simulink model "Gesamt"  (R2015b)
settings: Solver=ode3  SolverMode=SingleTasking  StartTime=0.0  StopTime=inf  RelTol=1e-3
InitFcn:
  | Reglerauslegung
values from neighbouring files (symbols this model uses):
  aMax = 498    [Reglerauslegung.m]
  aMaxPsi = 1    [Reglerauslegung.m]
  Blindzeit = 25    [Reglerauslegung.m]
  dt = 0.005    [Reglerauslegung.m]
  K1 = place(AI1,BI1,pWunschI1)    [Reglerauslegung.m]
  K2 = place(A2,B2,pWunsch2)    [Reglerauslegung.m]
  K3 = place(A3,B3,pWunsch3)    [Reglerauslegung.m]
  Kx = 0.9575    [Reglerauslegung.m]
  Ky = 0.9575    [Reglerauslegung.m]
  Tx = 1/4.1668    (= 0.239992320246)    [Reglerauslegung.m]
  Ty = 1/4.1668    (= 0.239992320246)    [Reglerauslegung.m]
  vMax = 403    [Reglerauslegung.m]
  vMaxPsi = 3    [Reglerauslegung.m]
undefined symbols (not defined in the file or in its folder): sigbuilder_block
libraries: simulink x5, xpcutilitieslib x1
(part 2 of 3)

== stateflow chart Gesamt/Bahnplanung1/Kommunikation_mit_GW1_3 ==
  settings: updateMethod=DISCRETE  sampleTime=dt
  state KommunikationGW3
    state Transportbereich
      entry:Transportbereich=1,
      Fertigungsbereich=0,
      Bereich_Verlassen=0,
      Status=1;
    state Fertigungsbereich
      entry:Transportbereich=0,
      Fertigungsbereich=1;
      state RFID_einchecken
        entry:Zielposition=Ziel-mod(Ziel,10)+3,
        Aktion_an_Position=Aktion_Warten,
        Status=2;
      state Startpunkt
        entry: Zielposition=Ziel-mod(Ziel,10);
        Aktion_an_Position=Aktion_Warten,
        Status=1;
      state Warten1
      state Warten
        during: Bereich_Verlassen=1,
      state Position_anfahren
        entry:Zielposition=Ziel,
        Status=1,
        if Werkstueck==0
        Aktion_an_Position=Aktion_Aufnehmen;
        else
        Aktion_an_Position=Aktion_Ablegen;
        end
      state Bereich_verlassen_vorne1
        entry:Zielposition=Ziel-mod(Ziel,10),
        Aktion_an_Position=Aktion_Warten,
        Status=1;
      state Bereich_verlassen_hinten
        entry:Zielposition=Ziel-mod(Ziel,10)+4,
        Aktion_an_Position=Aktion_Warten,
        Status=1;
      state Bereich_verlassen
        entry:
        ersterFifo=floor(floor(Ziel/10)/2)*3+2*mod(floor(Ziel/10),2)+1;
        Aktion_an_Position=Aktion_Warten,
      state RFID_auschecken
        entry:Zielposition=Ziel-mod(Ziel,10)+3,
        Aktion_an_Position=Aktion_Warten,
        Status=3;
      state Warten2
      Startpunkt -> RFID_einchecken [order 1] : [Ziel_anfordern==1 & Werkstueck==1]
      (default) -> Startpunkt
      RFID_einchecken -> Warten1 : [Ziel_anfordern==1 ]
      Startpunkt -> Position_anfahren [order 2] : [Ziel_anfordern==1 & Werkstueck==0]
      Warten1 -> Position_anfahren : [RFID_Anmeldung==1]
      Bereich_verlassen_vorne1 -> Warten : [Ziel_anfordern==1]
      Bereich_verlassen_hinten -> Warten : [Ziel_anfordern==1]
      Position_anfahren -> Bereich_verlassen [order 2] : [Ziel_anfordern==1 & (Aktion_an_Position==Aktion_Ablegen)]
      Position_anfahren -> RFID_auschecken [order 1] : [Ziel_anfordern==1 & (Aktion_an_Position==Aktion_Aufnehmen)]
      Bereich_verlassen -> Bereich_verlassen_vorne1 [order 1] : [FifoArray(ersterFifo)==0]
      Bereich_verlassen -> Bereich_verlassen_hinten [order 2]
      Warten2 -> Bereich_verlassen : [RFID_Abmeldung==1]
      RFID_auschecken -> Warten2 : [Ziel_anfordern==1]
    state Warten3
    state Ladestationanfahren
      entry:Transportbereich=0,
      Fertigungsbereich=1,
      Status=1;
    (default) -> Transportbereich
    Transportbereich -> Fertigungsbereich [order 1] : [(ZielStation_Erreicht==1) & (floor(Ziel/10)<=7)]
    Warten3 -> Transportbereich
    Transportbereich -> Ladestationanfahren [order 2] : [(ZielStation_Erreicht==1) & (floor(Ziel/10)>7)]
    Fertigungsbereich -> Warten3 : [Bereich_Verlassen==1]
  data: Transportbereich output; Fertigungsbereich output; Ziel input; Zielposition output; Aktion_an_Position output double; Aktion_Warten local double =0; Aktion_Aufnehmen local double =1; Aktion_Ablegen local double =2; Werkstueck input double; Bereich_Verlassen local; Status output; FifoArray input; ersterFifo local double; Ziel_anfordern input; ZielStation_Erreicht input double; RFID_Anmeldung input; RFID_Abmeldung input

== matlab function Gesamt/Bahnplanung1/Positionen_Robotinos_Filtern ==
  data: UDPDaten input; RobPos output; RobotinoID input; StoerPos output size=[1 15]; altePos input size=[1 15]; altePos1 output size=[1 15]
function [RobPos,StoerPos,altePos1]      = fcn(UDPDaten , RobotinoID, altePos)
StoerPos=zeros([1 15]);
RobPos=zeros([1 3]);
altePos1=zeros([1 15]);
%     case 5
%         RobPos(1:3) = UDPDaten(13:15);
%         StoerPos(1:12)=UDPDaten(1:12);
%Positionmerken
for x=0:4
    temp=abs(UDPDaten((x*3)+1:(x*3)+3));
    test=sum(temp);
    if(test==0)
     altePos1((x*3)+1:(x*3)+3)=altePos((x*3)+1:(x*3)+3);
    else
     altePos1((x*3)+1:(x*3)+3)=UDPDaten((x*3)+1:(x*3)+3);
    end
end

 if RobotinoID == 4
        RobPos(1:3) = altePos1(10:12);
        StoerPos(1:9)=altePos1(1:9);
        %  StoerPos(10:12)=UDPDaten(13:15);
    elseif RobotinoID == 3
        RobPos(1:3) = altePos1(7:9);
        StoerPos(1:6)=altePos1(1:6);
        StoerPos(7:9)=altePos1(10:12);%      StoerPos(7:12)=UDPDaten(10:15);
    elseif RobotinoID == 2
        RobPos(1:3) = altePos1(4:6);
        StoerPos(1:3)=altePos1(1:3);
        StoerPos(4:9)=altePos1(7:12);%     StoerPos(4:12)=UDPDaten(7:15);
        elseif RobotinoID == 1
        RobPos(1:3) = altePos1(1:3);
        StoerPos(1:9)=altePos1(4:12);%     StoerPos(1:12)=UDPDaten(4:15);
end

== matlab function Gesamt/Bahnplanung1/Trafo ==
  data: Vektor input; V_RobX output; Winkel input; V_RobY output
function [V_RobX, V_RobY]= fcn(Vektor,Winkel)
V_RobX=(cos(Winkel)*Vektor(1)+sin(Winkel)*Vektor(2));
V_RobY=(cos(Winkel)*Vektor(2)-sin(Winkel)*Vektor(1));

== matlab function Gesamt/Bahnplanung1/Vektorberechnung/AusweichVektorBerechnung ==
  data: Vektor_In input; Vektor output; Ausweichwert input; Zone input; RobotinoPos input; ZielPos input
function Vektor  = fcn(Vektor_In,Ausweichwert,Zone,RobotinoPos,ZielPos)
Vektor=zeros([1 2]);
%Ausweichmanöver
Distanz=sqrt((RobotinoPos(1)-ZielPos(1))^2+(RobotinoPos(2)-ZielPos(2))^2);
K=3;
AVX=zeros([1 4]);
AVY=zeros([1 4]);
 for x=1:4
 AVX(x)=-K*Ausweichwert(2,x)*cos(Ausweichwert(1,x));
 AVY(x)=-K*Ausweichwert(2,x)*sin(Ausweichwert(1,x));
 end
if (Zone==0) && ((Distanz > 300)&&(RobotinoPos(2)> 500)&&(RobotinoPos(1)> 500))
 VektorX=Vektor_In(1)+sum(AVX);
 VektorY=Vektor_In(2)+sum(AVY);
else
 VektorX=Vektor_In(1);
 VektorY=Vektor_In(2);
end

%Bremsen vor dem Ziel

MaxDis=1000;
if Distanz > MaxDis
Vektor(1) = VektorX;
Vektor(2) = VektorY;
else
Vektor(1) = VektorX*Distanz/MaxDis;
Vektor(2) = VektorY*Distanz/MaxDis;  
end

end

== matlab function Gesamt/Bahnplanung1/Vektorberechnung/Ausweichmanoever ==
  data: RobotinoPos input; StoerPos input; Vektor input; Ausweich output
function Ausweich  = fcn(RobotinoPos, StoerPos, Vektor)
Abstand=zeros([2 4]);
Ausweich=zeros([2 4]);%Zeile1 =Richtung(winkel in Rad) Zeile2=Intensität
for i=1:4
    Abstand(1,i)=-RobotinoPos(1)+StoerPos(1+((i-1)*3));
    Abstand(2,i)=-RobotinoPos(2)+StoerPos(2+((i-1)*3));
    Hyp=sqrt(Abstand(1,i)^2+Abstand(2,i)^2);
    if Hyp <=1000
        if Abstand(1,i) >= 0
             Ausweich(1,i)=+asin(Abstand(2,i)/Hyp)-pi/2;
        else
            Ausweich(1,i)=-asin(Abstand(2,i)/Hyp)+pi/2;
        end
        HypZiel=sqrt(Vektor(1)^2+Vektor(2)^2);
         if Vektor(1) >= 0
            Fahrwinkel=+asin(Vektor(2)/HypZiel);
        else
            Fahrwinkel=-asin(Vektor(2)/HypZiel)+pi;
        end
        if abs(Fahrwinkel-(Ausweich(1,i)+pi/2))<=pi
            if((Fahrwinkel-(Ausweich(1,i)+pi/2)) <= pi/6) && ((Fahrwinkel-(Ausweich(1,i)+pi/2))  >= -pi/6)
            Ausweich(2,i)=1;
             else
           Ausweich(2,i)=0; 
            end
        else
            if((2*pi)-abs(Fahrwinkel-(Ausweich(1,i)+pi/2)) <= pi/6) 
            Ausweich(2,i)=1;
             else
           Ausweich(2,i)=0; 
            end
        end
        if (abs(Fahrwinkel)>pi/2) && (RobotinoPos(2)>1900)
             if abs(Fahrwinkel-(Ausweich(1,i)+pi/2))<=pi
            if((Fahrwinkel-(Ausweich(1,i)+pi/2)) <= pi/6) && ((Fahrwinkel-(Ausweich(1,i)+pi/2))  >= -pi/6)
            Ausweich(2,i)=-1;
             else
           Ausweich(2,i)=0; 
            end
        else
            if((2*pi)-abs(Fahrwinkel-(Ausweich(1,i)+pi/2)) <= pi/6) 
            Ausweich(2,i)=-1;
             else
           Ausweich(2,i)=0; 
            end
        end
        end
%         if (Vektor(2)~=0) && (sin(Ausweich(1,i)+pi/2)~=0)
%             Ausweich(2,i)=Vektor(2)/sin(Ausweich(1,i)+pi/2);
%         elseif (Vektor(1)~=0)&&(cos(Ausweich(1,i)+pi/2)~=0)
%              Ausweich(2,i)=Vektor(1)/cos(Ausweich(1,i)+pi/2);
%         else
%              Ausweich(2,i)=0;
%         end
    else
        Ausweich(1,i)=0;
        Ausweich(2,i)=0;
    end
    if StoerPos(2+((i-1)*3))<300
        Ausweich(2,i)=0;
    end
end

== matlab function Gesamt/Bahnplanung1/Vektorberechnung/FahrendeRobotinosErkennen ==
  data: Stoerpos input; Robotinofaehrt output; Stoeralt input
function Robotinofaehrt = fcn(Stoerpos,Stoeralt)
Robotinofaehrt=zeros([1 4]);
for x=1:4
    if (abs(Stoeralt(1+(3*(x-1)))-Stoerpos(1+(3*(x-1)))) >= 10) && (abs(Stoeralt(2+(3*(x-1)))-Stoerpos(2+(3*(x-1)))) >= 10)
        Robotinofaehrt(x)=1;
    else
        Robotinofaehrt(x)=0;
    end
end

== matlab function Gesamt/Bahnplanung1/Vektorberechnung/IR_Daten_Erfassen ==
  data: RobotinoDaten input; IRWerte output; RobPos input
function IRWerte = fcn(RobotinoDaten,RobPos)
IRWerte=zeros([2 9]);
IRDaten=zeros([1 9]);
IRDaten=RobotinoDaten(6:14);

for x=1:9
    if  (isnan(IRDaten(x))==0) && (IRDaten(x) <= 120)
    IRWerte(1,x)=cos(((x-1)*40*pi/180)+RobPos(3))*(IRDaten(x)+200)+RobPos(1);
    IRWerte(2,x)=sin(((x-1)*40*pi/180)+RobPos(3))*(IRDaten(x)+200)+RobPos(2);
    else
    IRWerte(1,x)=NaN;
    IRWerte(2,x)=NaN;
    end
end

== matlab function Gesamt/Bahnplanung1/Vektorberechnung/Vektorberechnung ==
  data: ZielPos input; Vektor output; RobotinoPos input; StoerPos input; IRWerte input; Zone output; RobotinoFaehrt input; AlteZone input
function [Vektor,Zone] = fcn(ZielPos, RobotinoPos, StoerPos, IRWerte,RobotinoFaehrt,AlteZone)
Stationen=[1103,2308,3507,4694,6300,6300;
            2832,2832,2832,2832,2608,3085;];
Vektor=zeros([1 2]);
%Stationen Einflussvektor
K=400;
sigma=187;
SVX=zeros([1 6]);
SVY=zeros([1 6]);
for x=1:4
SVX(x)= -K*exp(-((RobotinoPos(1)-Stationen(1,x))^2+(RobotinoPos(2)-Stationen(2,x))^2)/(2*(sigma^2)))*((RobotinoPos(1)-Stationen(1,x))/(sigma^2));
SVY(x)= -K*exp(-((RobotinoPos(1)-Stationen(1,x))^2+(RobotinoPos(2)-Stationen(2,x))^2)/(2*(sigma^2)))*((RobotinoPos(2)-Stationen(2,x))/(sigma^2));
end
K=300;
sigma=100; %% mal schauen ob so gut
for x=5:6
SVX(x)= -K*exp(-((RobotinoPos(1)-Stationen(1,x))^2+(RobotinoPos(2)-Stationen(2,x))^2)/(2*(sigma^2)))*((RobotinoPos(1)-Stationen(1,x))/(sigma^2));
SVY(x)= -K*exp(-((RobotinoPos(1)-Stationen(1,x))^2+(RobotinoPos(2)-Stationen(2,x))^2)/(2*(sigma^2)))*((RobotinoPos(2)-Stationen(2,x))/(sigma^2));
end
%Zielvektor
K=0.5;%=0.3;

ZVX = K*(RobotinoPos(1)-ZielPos(1))/sqrt((RobotinoPos(1)-ZielPos(1))^2 +(RobotinoPos(2)-ZielPos(2))^2);
ZVY = K*(RobotinoPos(2)-ZielPos(2))/sqrt((RobotinoPos(1)-ZielPos(1))^2 +(RobotinoPos(2)-ZielPos(2))^2);

%Robtino Stoervektoren
%K=25 im Fifo

RVX=zeros([1 4]);
RVY=zeros([1 4]);
for x=1:4
if (RobotinoFaehrt(x) == 1) && (RobotinoPos(2)> 500)
K=1000;%K=100;
sigma=225;
elseif (RobotinoPos(2)> 2500)
K=500;
sigma=180;
elseif (RobotinoPos(2)< 2500)
K=700;
sigma=180;
end
RVX(x)=-K*exp(-((RobotinoPos(1)-StoerPos((x*3)-2))^2+(RobotinoPos(2)-StoerPos((x*3)-1))^2)/(2*(sigma^2)))*((RobotinoPos(1)-StoerPos((x*3)-2))/(sigma^2));
RVY(x)=-K*exp(-((RobotinoPos(1)-StoerPos((x*3)-2))^2+(RobotinoPos(2)-StoerPos((x*3)-1))^2)/(2*(sigma^2)))*((RobotinoPos(2)-StoerPos((x*3)-1))/(sigma^2));
end

%Infrarot Einflussvektor
K=500;
sigma=250;
IRVX=zeros([1 9]);
IRVY=zeros([1 9]);
for x=1:9
    if(isnan(IRWerte(1,x))==0)||(isnan(IRWerte(2,x))==0)
       if (RobotinoPos(2)> 500)
    IRVX(x)=-K*exp(-((RobotinoPos(1)-IRWerte(1,x))^2+(RobotinoPos(2)-IRWerte(2,x))^2)/(2*(sigma^2)))*((RobotinoPos(1)-IRWerte(1,x))/(sigma^2));
    IRVY(x)=-K*exp(-((RobotinoPos(1)-IRWerte(1,x))^2+(RobotinoPos(2)-IRWerte(2,x))^2)/(2*(sigma^2)))*((RobotinoPos(2)-IRWerte(2,x))/(sigma^2));
       else
    IRVX=0;
    IRVY=0;
       end
    else
    IRVX(x)=0;
    IRVY(x)=0;
    end
end


 
K=0.4; %Steigung der schrägen
x=RobotinoPos(1);
y=RobotinoPos(2);
x_test=0;
y_test=0;
VektorX=0;
VektorY=0;

 if (x >601) && (x<=5301) && (y>2501) && (y<=3201)
    Zone=4;
elseif (x >2751) && (x<=5501) && (y>3201)
    Zone=1;
elseif (x > 601) && (x<=2751) && (y>3201)
    Zone=2;
 elseif (x<=601) && (y>2501)
     Zone=3;  
 elseif (x >5001) && (y>2501) && (AlteZone==1 || AlteZone==5)
     Zone=5;
 else
     Zone=0;
 end

KE=1000;
sigma=50;
Parabel=1000;
 if Zone == 0 % Fahrbereich
     if (x <= 5500) && (y <= 2500)
         x_test=(1/sigma)*KE*exp(-x/sigma);
         y_test=(-1/sigma)*KE*exp((y-2500)/sigma);
     elseif (x > 5500) && (y <= 2500)
         x_test=(1/sigma)*KE*exp((-(x-5500)+(y-2500))/sigma);
         y_test=(-1/sigma)*KE*exp((-(x-5500)+(y-2500))/sigma);
     elseif (x > 5500) && (y > 2500)
         x_test=(1/sigma)*KE*exp(-(x-5500)/sigma);
         y_test=(-1/sigma)*KE*exp((y-3600)/sigma);
     end
 MVX=x_test+(-1/sigma)*KE*exp((x-7000)/sigma);
 MVY=y_test+(1/sigma)*KE*exp(-y/sigma);
 
 VektorX=sum(SVX(5:6))+sum(RVX)+ZVX+sum(IRVX)-MVX;
 VektorY=sum(SVY(5:6))+sum(RVY)+ZVY+sum(IRVY)-MVY;
 elseif Zone == 1 %Rinne nach rechts weg
     MVX=K; %Konstante Steigung
     MVY=-2*(y-3500)/Parabel; % Parabel abgeleitet
 VektorX=sum(RVX)-MVX;
 VektorY=sum(RVY)-MVY;
 elseif Zone == 2 %Rinne nach links weg
     MVX=-K; %Konstante Steigung
     MVY=-2*(y-3500)/Parabel; % Parabel abgeleitet
      VektorX=sum(RVX)-MVX;
      VektorY=sum(RVY)-MVY;
 elseif Zone == 3 %Rinne nach unten weg
     MVX=-2*(x-300)/Parabel; %Konstante Steigung
     MVY=-K; % Parabel abgeleitet
     VektorX=sum(RVX)+sum(IRVX)-MVX;
     VektorY=sum(RVY)+sum(IRVY)-MVY;
 elseif Zone == 5 %Rinne vorne weg
     MVX=-2*(x-5500)/Parabel; %Konstante Steigung
     MVY=-K; % Parabel abgeleitet
     VektorX=sum(RVX)+sum(IRVX)-MVX;
     VektorY=sum(RVY)+sum(IRVY)-MVY;
 else 
     MVX=0;
     MVY=K;
      VektorX=sum(RVX)+sum(SVX(1:4))-MVX;
      VektorY=sum(RVY)+sum(SVY(1:4))-MVY;
 end  
      Vektor(1)=VektorX;
      Vektor(2)=VektorY;
 end

== matlab function Gesamt/Bahnplanung1/Fifo Steuerung/Globale Markierung1 ==
  data: Robbi input; FifoArray input; FifoArray1 output; StationArray1 output; LadeArray input; LadeArray1 output
function [FifoArray1,StationArray1,LadeArray1]= fcn(Robbi,FifoArray,LadeArray)
X=zeros([1 4]);
Y=zeros([1 4]);
X=[Robbi(1) Robbi(4) Robbi(7) Robbi(10)];
Y=[Robbi(2) Robbi(5) Robbi(8) Robbi(11)];
FifoArray1=zeros([1 12]);
FifoArray1=FifoArray(1:12);
StationArray1=zeros([1 8]);
LadeArray1=zeros([1 2]);
LadeArray1=LadeArray(1:2);
N=zeros([1 4]);
S=zeros([1 4]);
L=zeros([1 4]);
for n= 1 : 1 : 4
    L(n)=round((Y(n)-2592)/500)+1;
    N(n)=round((X(n)-703)/400)+1;   % Berechnung in welchem Fifo der Roboter sich befindet
    S(n)=round((X(n)-900)/560)+1;   %Berechnung in welcher Station der Roboter sich befindet
     if (X(n)<=6000 || X(n)>6500)
        for i=1:2
            if LadeArray1(i)==n
                LadeArray1(i)=0;
            end
        end
     end
    if (X(n)>6000 && X(n)<=6500 && Y(n)>2300 && Y(n)<=3300)
        LadeArray1(L(n))=n;
    end  
   
    for i=1:8
          if StationArray1(i)==n
                StationArray1(i)=0;
          end
    end
    if (Y(n)>2100 && Y(n)<3300 && X(n)<5100) && S(n)<=8 && S(n)>0
         for i=1:12
            if FifoArray1(i)==n
                FifoArray1(i)=0;
            end
         end
       
        StationArray1(S(n))=n;
        
    elseif (Y(n)<450 && (X(n)>100 && X(n)<5250)&& N(n)<=12 && N(n)>0)
        for i=1:12
            if FifoArray1(i)==n
                FifoArray1(i)=0;
            end
        end
            FifoArray1(N(n))=n;
           
    elseif (X(n)>6000&& Y(n)<2000)
        for i=1:12
            if FifoArray1(i)==n
                FifoArray1(i)=0;
            end
        end
    end
    end
end

== matlab function Gesamt/Bahnplanung1/Vektorbrbegrenzungberchnen1 ==
  data: Vektor_In input; Vektor output; Transportbereich_aktiv input; RobPos input; FilterIN input; Filter output
function [Vektor,Filter] = fcn(Vektor_In,Transportbereich_aktiv,RobPos,FilterIN)
Vektor=zeros([1 2]);
Filter=zeros([100 2]);
if (Transportbereich_aktiv==1) && (RobPos(1)>=0) && (RobPos(2)>=0)
    

 Filter(1,1)=Vektor_In(1);
 Filter(1,2)=Vektor_In(2);
 for x=1:99
     Filter(x+1,1)=FilterIN(x,1);
     Filter(x+1,2)=FilterIN(x,2);     
 end
 Vektor(1) =sum(Filter(:,1))/100;
 Vektor(2) =sum(Filter(:,2))/100;
 
 %Vektor(1) = Vektor_In(1);
 %Vektor(2) = Vektor_In(2);

if (RobPos(2)<500)||(RobPos(2)>2300)
    for x=1:2
    K=0.3; %Begrenzung langsame Zone
        if  Vektor(x)> K
            Vektor(x) = K;
        elseif Vektor(x) <-K
            Vektor(x)=-K;
        end
    end
else
    for x=1:2
    K=0.5; %Begrenzung schnelle Zone
        if  Vektor(x)> K
            Vektor(x) = K;
        elseif Vektor(x) <-K
            Vektor(x)=-K;
        end
    end
end
end

== matlab function Gesamt/Regelung1/Kalman1 ==
  data: vxZustand input; vyZustand input; vPsiZustand input; PsiZustand input; xZustand input; yZustand input; enable input; dt parameter; vx output; vy output; vpsi output; pospsi output; posx output; posy output; enableBeob output; Blindzeit parameter
function [vx,vy,vpsi,pospsi,posx,posy,enableBeob] = fcn(vxZustand,vyZustand,vPsiZustand,PsiZustand,xZustand,yZustand,enable,dt,Blindzeit)

persistent A H Q RPosX RPosY RPosPsi 
persistent x P
persistent firstRun found counter
QVelX = 0.01;
QVelY = 0.01;
QVelPsi = 0.01;
QPosX = 0.01;
QPosY = 0.01;
QPosPsi = 0.1;
if isempty(firstRun)
found = 0;
x = [0; 0; 0; 0; 2000; 1600];
    

A= [1       0       0       0       0       0;
    0       1       0       0       0       0;
    0       0       1       0       0       0;
    0       0       dt      1       0       0;
    dt      0       0       0       1       0;
    0       dt      0       0       0       1];
    
H = [0 0 0 1 0 0;
     0 0 0 0 1 0;
     0 0 0 0 0 1];

Q = [QVelX       0       0       0       0       0;
     0       QVelY       0       0       0       0;
     0          0       QVelPsi    0       0       0;
     0          0       0       QPosX    0       0;
     0          0       0       0       QPosY    0;
     0          0       0       0       0    QPosPsi];
   
  RPosX = 0.340050836575258;
  RPosY =0.684587581598845;
  RPosPsi=5.754253525875726e-05;

  P =  [1       0       0       0       0       0;
        0       1       0       0       0       0;
        0       0       1       0       0       0;
        0       0       0       1000       0       0;
        0       0       0       0       1000       0;
        0       0       0       0       0       1000];
  
  firstRun = 1; 
  counter = 0;
end


x =[vxZustand ; vyZustand; vPsiZustand;x(4:end,1)];

x = A*x;  
P = A*P*A' + Q;  
counter = counter+1;
dist=0;
Rnow=[RPosX 0 0; 0 RPosY 0; 0 0 RPosPsi];
if enable == 1
    z = [PsiZustand;xZustand;yZustand];
    % Reduzierung der Glaubwürdigkeit bei weit entfernten Messungen
    dist = sqrt(abs(z(2)-x(5))^2 + abs(z(3)-x(6))^2);
    counter =0;
    
%     if dist > 150
%         Rnow = 0;
%         found = 0;
%     elseif dist > 100
%         Rnow = 0.3;
%         found = 0;
%     elseif dist > 20
%         Rnow = 0.2;
%         found = 1;
%     elseif dist < 20
%         found =1;
%         Rnow = 0.5;
%     else 
%         Rnow = R;
%     end

%     if dist > 500
%         Rnow = 0;
%         found = 0;
%     elseif dist > 100
%         Rnow = 0;
%         found = 0;
%     elseif dist > 20
%         Rnow = 0;
%         found = 1;
%     elseif dist < 20
%         found =1;
%         Rnow = 0;
%     else 
%         Rnow = R;
%     end

%     if dist > 500
%         Rnow = eye(3,3)*0;
%         found = 0;
%     elseif dist > 100
%         Rnow=[RPosX-0.1 0 0; 0 RPosY-0.1 0; 0 0 RPosPsi-0.01];
%         found = 0;
%     elseif dist > 20
%         Rnow=[RPosX-0.01 0 0; 0 RPosY-0.01 0; 0 0 RPosPsi];
%         found = 1;
%     else 
%         found = 1;
%         Rnow=[RPosX 0 0; 0 RPosY 0; 0 0 RPosPsi];
%     end
    if dist > 20
        found = 1;
    end
    K =    P*H'*inv(H*P*H' + Rnow); 

    x = x + K*(z - H*x);

    P = P - K*H*P;
end
if counter>= (Blindzeit/dt)
    found = 0;
end
enableBeob = found;

vx      = x(1);
vy      = x(2);
vpsi    = x(3);
pospsi  = x(4);
posx    = x(5);
posy    = x(6);

== matlab function Gesamt/Regelung1/Bereichswaehler ==
  data: modus output; transportbereich input; enable output; fertigungsbereich input
function [modus, enable] = fcn(transportbereich, fertigungsbereich)

enable = false;
modus = 0;

if fertigungsbereich == 1 && transportbereich == 0
    enable = true;
    modus = 1;
end
    
if fertigungsbereich == 0 && transportbereich == 1
    enable = true;
    modus = 0;
end

== matlab function Gesamt/Regelung1/NewCam ==
  data: yZustand input; xZustand input; psiZustand input; enable output
function enable = fcn(yZustand,xZustand,psiZustand)


persistent oldx oldy oldpsi firstRun

if isempty(firstRun)
   firstRun = 1;
   oldx     = -1;
   oldy     = -1;
   oldpsi   = -1;
   firstRun = 2;
end

if ( xZustand == 0 && yZustand == 0)
    firstRun = 1;
    enable = 0;
elseif firstRun < 2
    firstRun = firstRun +1;
    enable =0;
else  
    if((mod(firstRun,1) == 0)&&((oldx ~= xZustand) || (oldy ~= yZustand) || (oldpsi ~= psiZustand)))
        enable = 1;
       oldx     = xZustand;
       oldy     = yZustand;
       oldpsi   = psiZustand;

    else
        enable = 0;
    end
end

== matlab function Gesamt/Regelung1/Receiver/autoRobID ==
  data: udpIn input; pX output; pY output; psi output; enable output; robID input
function [pX, pY, psi, enable] = autoRobID(udpIn, robID)
enable  = 1;
pX      = 0;
pY      = 0;
psi     = 0;

if robID == 1
    pX      = udpIn(1);
    pY      = udpIn(2);
    psi     = udpIn(3);
elseif robID == 2
    pX      = udpIn(4);
    pY      = udpIn(5);
    psi     = udpIn(6);
elseif robID == 3
    pX      = udpIn(7);
    pY      = udpIn(8);
    psi     = udpIn(9);
elseif robID == 4
    pX      = udpIn(10);
    pY      = udpIn(11);
    psi     = udpIn(12);
elseif robID == 5
    pX      = udpIn(13);
    pY      = udpIn(14);
    psi     = udpIn(15);
end

if (pX == 0) && (pY == 0)
    enable = 0;
end

== matlab function Gesamt/Regelung1/Receiver/x4(psi) ==
  data: psi input; x4 output
function x4 = Winkelkorrektur(psi)

persistent turnCounter firstRun lastAngle

if isempty(firstRun)
    firstRun = 1;
    turnCounter = 0;
    lastAngle = 0;
end

% Kamera gibt uns -pi bis + pi
% Wir wollen 0 bis 2pi
psi = mod(psi+2*pi,2*pi);

% winkel kontinuierlich hoch bzw runterzaehlen
if( (psi < (2*pi)/5) && (lastAngle > ((2*pi) - (2*pi)/5) ) )
    turnCounter = turnCounter + 1;
end

if( (lastAngle < (2*pi)/5) && (psi > ((2*pi) - (2*pi)/5) ) )
    turnCounter = turnCounter - 1;
end

lastAngle = psi;

x4 = psi + turnCounter * 2*pi;

== matlab function Gesamt/Regelung1/Robotino interface/assemble robotino response ==
  data: v_x_in input; robotino_response output; v_y_in input; v_theta_in input; distance_measuring_sensors_in input; bumper_in input; light_barrier_in input; slider_in input
%%%%%%%%%%%%%%%%%%%%%%%%%%%%%%%%%%%%%%%%%%%%%%%%%%%%%%%%%%%%%%%%%%%%%%%%%%%
% Assembly of robot data in a vector of 34 elements.                      %
%                                                                         %
% inputs:   longitudinal, lateral and rotational velocity (in mm/s),      %
%           shaft positions of the three motors (4 elements per motor),   %
%           running times of the three motors (3 elements per motor),     %
%           values of the nine IR-sensors (in mm),                        %
%           bumper collision (1 = no collision;                           %
%                             0 = collision)                              %
% outputs:  vector containing assembled input data                        %
%%%%%%%%%%%%%%%%%%%%%%%%%%%%%%%%%%%%%%%%%%%%%%%%%%%%%%%%%%%%%%%%%%%%%%%%%%%
function robotino_response = fcn(v_x_in, v_y_in, v_theta_in, ...
                                 distance_measuring_sensors_in, ...
                                 bumper_in, light_barrier_in, slider_in)
                                 % motor_positions_in, time_bytes_in, ...)
robotino_response = [light_barrier_in, slider_in, v_x_in, v_y_in, ...
                     v_theta_in, ...%motor_positions_in, time_bytes_in, ...
                     distance_measuring_sensors_in', bumper_in]';

== matlab function Gesamt/Regelung1/Stellgrößen- beschränkung /Beschraenkung  ==
  data: MaxStellT input; MaxStellR input; x input; X output; Y output; y input; theta input; Theta output; enableGewerk3 input
function [X,Y,Theta] = Beschraenkung(MaxStellT,MaxStellR,x,y,theta,enableGewerk3)

if (x > MaxStellT)
    X = MaxStellT;
elseif  (x < -MaxStellT)
    X = -MaxStellT;
else 
    X = x;
end

if (y > MaxStellT)
    Y = MaxStellT;
elseif  (y < -MaxStellT)
    Y = -MaxStellT;
else
    Y = y;
end

if (theta > MaxStellR)
    Theta = MaxStellR;
elseif  (theta < -MaxStellR)
    Theta = -MaxStellR;
else
    Theta = theta;
end

if enableGewerk3 == 0
    X = 0;
    Y = 0;
    Theta = 0;
end

== matlab function Gesamt/Regelung1/Zustandsautomat/Bahnplanung Psi ==
  settings: updateMethod=DISCRETE  sampleTime=dt
  data: zielPosition input; istPosition input; enable input; sollPosition output; dt parameter; sollGeschwindigkeit output; aMaxPsi parameter; vMaxPsi parameter
% s = 1/2 * m * t^2
% v = m * t
% a = m

function [sollPosition, sollGeschwindigkeit]= Bahnplanung(zielPosition,istPosition,enable,dt,aMaxPsi,vMaxPsi)
    
%     aMax = 0.5;  % Maximale Beschleunigung
%     vMax = 2; % Maximale Geschwindigkeit
     nGr = 1000; % Groesse der Planvektoren

    persistent firstRun s v nZyklen nZyklenK fertig  n
    
    if isempty(firstRun)
        firstRun = 1;
        s = 0;          % Vektor mit Wegdaten
        v = 0;          % Vektor mit Geschwindigkeitsdaten
        nZyklen = 0;    % Anzahl der benoetigten Zyklen
        nZyklenK = 0;
        n = 1;          % Zaehlvariable
        fertig = 0;
    end

    if (enable == 1) || (fertig == 1)
        n = 1;
        Out = 1;
        startPosition = mod(istPosition,2*pi);
        % Berechnung der optimalen Drehrichtung
        
        if (abs(zielPosition-startPosition) <= pi)   % (1)
    
            Out = zielPosition - startPosition;      % (2)

        else

             if (zielPosition > startPosition)                % (3)
                Out = zielPosition - startPosition - 2*pi;    % (4)
             else
                 Out = zielPosition - startPosition + 2*pi;   % (5)
             end
        end
        
        % Berechnung der Zeitabschnitte für anfahren, konstant Fahren und bremsen
        tvMax   = 1/aMaxPsi * vMaxPsi ;       % Zeit bis maximale Geschw.(vMax) erreicht ist
        svMax   = 1/2 * aMaxPsi * tvMax^2; % Weg der zurueckgelegt wurde bis tvMax
        tK      = (abs(Out) - 2 * svMax) / vMaxPsi; % Zeit waehrend konstant gefahren wird
        % Fuer nur Anfahren und Bremsen
        tHalbe = sqrt(2 * 1/aMaxPsi * abs(Out)/2); % Zeit bis zur halben Strecke

        tBB = zeros(1,nGr);
        tBA = zeros(1,nGr);
        tBK = zeros(1,nGr);
        sA  = zeros(1,nGr);
        vA  = zeros(1,nGr);
        sB  = zeros(1,nGr);
        vB  = zeros(1,nGr);
        sK  = zeros(1,nGr);
        vK  = zeros(1,nGr);
        s   = zeros(1,3*nGr);
        v   = zeros(1,3*nGr);
        
        
        % Nur Anfahren und Bremsen
         if tvMax > tHalbe
            % Beschleunigung/Anfahrt
            nZyklen = ceil(tHalbe/dt);
            nZyklenK = 0;
            if nZyklen > nGr
                nZyklen = nGr;
            elseif nZyklen <= 0
                nZyklen = 1;
            end
            
            tBA(1:nZyklen) = linspace(0,tHalbe,nZyklen);%0:dt:(nZyklen)*dt-dt;

            sA(1:nZyklen) = sign(Out) * 1/2 * aMaxPsi * tBA(1:nZyklen).^2;
            vA(1:nZyklen) = sign(Out) *aMaxPsi * tBA(1:nZyklen);
            if sA(nZyklen) == 0
                offset = 1;
            else
                offset = 0;
            end
            % Bremsen
            tBB(1:nZyklen) = linspace(-tHalbe,0,nZyklen);%-nZyklen*dt+dt:dt:0;

            sB(1:nZyklen) = -sign(Out) * 1/2 * aMaxPsi * tBB(1:nZyklen) .^2 + 2*sA(nZyklen-offset);
            vB(1:nZyklen) = -sign(Out) * aMaxPsi * tBB(1:nZyklen);
            s(1:2*nZyklen) = [sA(1:nZyklen) sB(1:nZyklen)]+startPosition;
            v(1:2*nZyklen) = [vA(1:nZyklen) vB(1:nZyklen)];
            
        else
            % Beschleunigung/Anfahrt

            nZyklen = ceil((tvMax)/dt);
            nZyklenK = ceil(tK/dt);

            if nZyklen > nGr
                nZyklen = nGr;
            elseif nZyklen <= 0
                nZyklen = 1;
            end
            if nZyklenK > nGr
                nZyklenK = nGr;
            elseif nZyklenK <= 0
                nZyklenK = 1;
            end
            
            tBA(1:nZyklen) = linspace(0,tvMax,nZyklen);%0:dt:(nZyklen)*dt-dt;

            sA(1:nZyklen) = sign(Out) * 1/2 * aMaxPsi * tBA(1:nZyklen).^2;
            vA(1:nZyklen) = sign(Out) * aMaxPsi * tBA(1:nZyklen);
            if sA(nZyklen) == 0
                offset = 1;
            else
                offset = 0;
            end
            % Fahrt mit konstanter Geschwindigkeit
            tBK(1:nZyklenK) = linspace(0,tK,nZyklenK);%0:dt:(nZyklenK)*dt-dt;
            vK(1:nZyklenK)   = sign(Out) * vMaxPsi * ones(1,nZyklenK);
            sK(1:nZyklenK)   = sign(Out) * vMaxPsi * tBK(1:nZyklenK) + sA(nZyklen-offset);
            if sK(nZyklenK) == 0
                offsetK = 1;
            else
                offsetK = 0;
            end
            % Bremsen
            tBB(1:nZyklen) = linspace(-tvMax,0,nZyklen);%-(nZyklen)*dt+dt:dt:0;

            sB(1:nZyklen) = -sign(Out) *  1/2 * aMaxPsi * tBB(1:nZyklen).^2 + sA(nZyklen-offset)+sK(nZyklenK-offsetK);
            vB(1:nZyklen) = -sign(Out) *  aMaxPsi * tBB(1:nZyklen);
            s(1:2*nZyklen+nZyklenK) = [sA(1:nZyklen) sK(1:nZyklenK) sB(1:nZyklen)]+startPosition;
            v(1:2*nZyklen+nZyklenK) = [vA(1:nZyklen) vK(1:nZyklenK) vB(1:nZyklen)];
         end
        firstRun = 0;
    end
    % Ausgabe
    sollPosition = s(n);
    sollGeschwindigkeit = v(n);
    if n < (2*nZyklen+nZyklenK-1)
        n = n + 1;
         fertig = 0;
     elseif nZyklen == nGr || nZyklenK == nGr 
         fertig = 1;
    end

== matlab function Gesamt/Regelung1/Zustandsautomat/Bahnplanung X ==
  settings: updateMethod=DISCRETE  sampleTime=dt
  data: zielPosition input; istPosition input; enable input; sollPosition output; dt parameter; sollGeschwindigkeit output; aMax parameter; vMax parameter
% s = 1/2 * m * t^2
% v = m * t
% a = m

function [sollPosition, sollGeschwindigkeit]= Bahnplanung(zielPosition,istPosition,enable,dt,aMax,vMax)
    
%     aMax = 300;  % Maximale Beschleunigung
%     vMax = 500; % Maximale Geschwindigkeit
     nGr = 1000; % Groesse der Planvektoren

    persistent firstRun s v nZyklen nZyklenK fertig  n
    
    if isempty(firstRun)
        firstRun = 1;
        s = 0;          % Vektor mit Wegdaten
        v = 0;          % Vektor mit Geschwindigkeitsdaten
        nZyklen = 0;    % Anzahl der benoetigten Zyklen
        nZyklenK = 0;
        n = 1;          % Zaehlvariable
        fertig = 0;
    end

    if (enable == 1) || (fertig == 1)
        n = 1;
        startPosition = istPosition;
        % Berechnung der Zeitabschnitte für anfahren, konstant Fahren und bremsen
        tvMax   = 1/aMax * vMax ;       % Zeit bis maximale Geschw.(vMax) erreicht ist
        svMax   = 1/2 * aMax * tvMax^2; % Weg der zurueckgelegt wurde bis tvMax
        tK      = (abs(zielPosition-startPosition) - 2 * svMax) / vMax; % Zeit waehrend konstant gefahren wird
        % Fuer nur Anfahren und Bremsen
        tHalbe = sqrt(2 * 1/aMax * abs(zielPosition-startPosition)/2); % Zeit bis zur halben Strecke

        tBB = zeros(1,nGr);
        tBA = zeros(1,nGr);
        tBK = zeros(1,nGr);
        sA  = zeros(1,nGr);
        vA  = zeros(1,nGr);
        sB  = zeros(1,nGr);
        vB  = zeros(1,nGr);
        sK  = zeros(1,nGr);
        vK  = zeros(1,nGr);
        s   = zeros(1,3*nGr);
        v   = zeros(1,3*nGr);
%         % Nur Anfahren und Bremsen
         if tvMax > tHalbe
            % Beschleunigung/Anfahrt
            nZyklen = ceil(tHalbe/dt);
            nZyklenK = 0;
            if nZyklen > nGr
                nZyklen = nGr;
            elseif nZyklen <= 0
                nZyklen = 1;
            end
            
            tBA(1:nZyklen) = linspace(0,tHalbe,nZyklen);%0:dt:(nZyklen)*dt-dt;

            sA(1:nZyklen) = sign(zielPosition-startPosition) * 1/2 * aMax * tBA(1:nZyklen).^2;
            %sA(sA==0) = [];
            vA(1:nZyklen) = sign(zielPosition-startPosition) *aMax * tBA(1:nZyklen);
            % Bremsen
            tBB(1:nZyklen) = linspace(-tHalbe,0,nZyklen);%-nZyklen*dt+dt:dt:0;
            
            %manchmal klappt das mit dem runden nicht so gut...
            if sA(nZyklen) == 0
                offset = 1;
            else
                offset = 0;
            end
            
            sB(1:nZyklen) = -sign(zielPosition-startPosition) * 1/2 * aMax * tBB(1:nZyklen) .^2 + 2*sA(nZyklen-offset);
            vB(1:nZyklen) = -sign(zielPosition-startPosition) * aMax * tBB(1:nZyklen);
            s(1:2*nZyklen) = [sA(1:nZyklen) sB(1:nZyklen)]+startPosition;
            v(1:2*nZyklen) = [vA(1:nZyklen) vB(1:nZyklen)];
            
        else
            % Beschleunigung/Anfahrt

            nZyklen = ceil((tvMax)/dt);
            nZyklenK = ceil(tK/dt);

            if nZyklen > nGr
                nZyklen = nGr;
            elseif nZyklen <= 0
                nZyklen = 1;
            end
            if nZyklenK > nGr
                nZyklenK = nGr;
            elseif nZyklenK <= 0
                nZyklenK = 1;
            end
            
            tBA(1:nZyklen) = linspace(0,tvMax,nZyklen);%0:dt:(nZyklen)*dt-dt;

            sA(1:nZyklen) = sign(zielPosition-startPosition) * 1/2 * aMax * tBA(1:nZyklen).^2;
            vA(1:nZyklen) = sign(zielPosition-startPosition) * aMax * tBA(1:nZyklen);
            %manchmal klappt das mit dem runden nicht so gut...
            if sA(nZyklen) == 0
                offset = 1;
            else
                offset = 0;
            end
            % Fahrt mit konstanter Geschwindigkeit
            tBK(1:nZyklenK) = linspace(0,tK,nZyklenK);%0:dt:(nZyklenK)*dt-dt;
            vK(1:nZyklenK)   = sign(zielPosition-startPosition) * vMax * ones(1,nZyklenK);
            
            % wieso wir hier im gegensatz zu sB nur einmal sA
            % draufgerechnet statt 2*sA ?
            sK(1:nZyklenK)   = sign(zielPosition-startPosition) * vMax * tBK(1:nZyklenK) + sA(nZyklen-offset);
            
            if sK(nZyklenK) == 0
                offsetK = 1;
            else
                offsetK = 0;
            end
            % Bremsen
            tBB(1:nZyklen) = linspace(-tvMax,0,nZyklen);%-(nZyklen)*dt+dt:dt:0;
            %sB(1:nZyklen) = -sign(zielPosition-startPosition) * 1/2 * aMax * tBB(1:nZyklen) .^2 + 2*sA(nZyklen-offset);
            sB(1:nZyklen) = -sign(zielPosition-startPosition) *  1/2 * aMax * tBB(1:nZyklen).^2 + sA(nZyklen-offset)+sK(nZyklenK-offsetK);
            vB(1:nZyklen) = -sign(zielPosition-startPosition) *  aMax * tBB(1:nZyklen);
            s(1:2*nZyklen+nZyklenK) = [sA(1:nZyklen) sK(1:nZyklenK) sB(1:nZyklen)]+startPosition;
            v(1:2*nZyklen+nZyklenK) = [vA(1:nZyklen) vK(1:nZyklenK) vB(1:nZyklen)];
         end
        firstRun = 0;
    end
    % Ausgabe
    sollPosition = s(n);
    sollGeschwindigkeit = v(n);
    if n < (2*nZyklen+nZyklenK-1)
        n = n + 1;
         fertig = 0;
     elseif nZyklen == nGr || nZyklenK == nGr 
         fertig = 1;
    end

== matlab function Gesamt/Regelung1/Zustandsautomat/Bahnplanung Y ==
  settings: updateMethod=DISCRETE  sampleTime=dt
  data: zielPosition input; istPosition input; enable input; sollPosition output; dt parameter; sollGeschwindigkeit output; aMax parameter; vMax parameter
% s = 1/2 * m * t^2
% v = m * t
% a = m

function [sollPosition, sollGeschwindigkeit]= Bahnplanung(zielPosition,istPosition,enable,dt,aMax,vMax)
    
%     aMax = 300;  % Maximale Beschleunigung
%     vMax = 500; % Maximale Geschwindigkeit
     nGr = 1000; % Groesse der Planvektoren

    persistent firstRun s v nZyklen nZyklenK fertig  n
    
    if isempty(firstRun)
        firstRun = 1;
        s = 0;          % Vektor mit Wegdaten
        v = 0;          % Vektor mit Geschwindigkeitsdaten
        nZyklen = 0;    % Anzahl der benoetigten Zyklen
        nZyklenK = 0;
        n = 1;          % Zaehlvariable
        fertig = 0;
    end

    if (enable == 1) || (fertig == 1)
        n = 1;
        startPosition = istPosition;
        % Berechnung der Zeitabschnitte für anfahren, konstant Fahren und bremsen
        tvMax   = 1/aMax * vMax ;       % Zeit bis maximale Geschw.(vMax) erreicht ist
        svMax   = 1/2 * aMax * tvMax^2; % Weg der zurueckgelegt wurde bis tvMax
        tK      = (abs(zielPosition-startPosition) - 2 * svMax) / vMax; % Zeit waehrend konstant gefahren wird
        % Fuer nur Anfahren und Bremsen
        tHalbe = sqrt(2 * 1/aMax * abs(zielPosition-startPosition)/2); % Zeit bis zur halben Strecke

        tBB = zeros(1,nGr);
        tBA = zeros(1,nGr);
        tBK = zeros(1,nGr);
        sA  = zeros(1,nGr);
        vA  = zeros(1,nGr);
        sB  = zeros(1,nGr);
        vB  = zeros(1,nGr);
        sK  = zeros(1,nGr);
        vK  = zeros(1,nGr);
        s   = zeros(1,3*nGr);
        v   = zeros(1,3*nGr);
%         % Nur Anfahren und Bremsen
         if tvMax > tHalbe
            % Beschleunigung/Anfahrt
            nZyklen = ceil(tHalbe/dt);
            nZyklenK = 0;
            if nZyklen > nGr
                nZyklen = nGr;
            elseif nZyklen <= 0
                nZyklen = 1;
            end
            
            tBA(1:nZyklen) = linspace(0,tHalbe,nZyklen);%0:dt:(nZyklen)*dt-dt;

            sA(1:nZyklen) = sign(zielPosition-startPosition) * 1/2 * aMax * tBA(1:nZyklen).^2;
            %sA(sA==0) = [];
            vA(1:nZyklen) = sign(zielPosition-startPosition) *aMax * tBA(1:nZyklen);
            % Bremsen
            tBB(1:nZyklen) = linspace(-tHalbe,0,nZyklen);%-nZyklen*dt+dt:dt:0;
            
            %manchmal klappt das mit dem runden nicht so gut...
            if sA(nZyklen) == 0
                offset = 1;
            else
                offset = 0;
            end
            
            sB(1:nZyklen) = -sign(zielPosition-startPosition) * 1/2 * aMax * tBB(1:nZyklen) .^2 + 2*sA(nZyklen-offset);
            vB(1:nZyklen) = -sign(zielPosition-startPosition) * aMax * tBB(1:nZyklen);
            s(1:2*nZyklen) = [sA(1:nZyklen) sB(1:nZyklen)]+startPosition;
            v(1:2*nZyklen) = [vA(1:nZyklen) vB(1:nZyklen)];
            
        else
            % Beschleunigung/Anfahrt

            nZyklen = ceil((tvMax)/dt);
            nZyklenK = ceil(tK/dt);

            if nZyklen > nGr
                nZyklen = nGr;
            elseif nZyklen <= 0
                nZyklen = 1;
            end
            if nZyklenK > nGr
                nZyklenK = nGr;
            elseif nZyklenK <= 0
                nZyklenK = 1;
            end
            
            tBA(1:nZyklen) = linspace(0,tvMax,nZyklen);%0:dt:(nZyklen)*dt-dt;

            sA(1:nZyklen) = sign(zielPosition-startPosition) * 1/2 * aMax * tBA(1:nZyklen).^2;
            vA(1:nZyklen) = sign(zielPosition-startPosition) * aMax * tBA(1:nZyklen);
            %manchmal klappt das mit dem runden nicht so gut...
            if sA(nZyklen) == 0
                offset = 1;
            else
                offset = 0;
            end
            % Fahrt mit konstanter Geschwindigkeit
            tBK(1:nZyklenK) = linspace(0,tK,nZyklenK);%0:dt:(nZyklenK)*dt-dt;
            vK(1:nZyklenK)   = sign(zielPosition-startPosition) * vMax * ones(1,nZyklenK);
            sK(1:nZyklenK)   = sign(zielPosition-startPosition) * vMax * tBK(1:nZyklenK) + sA(nZyklen-offset);
            if sK(nZyklenK) == 0
                offsetK = 1;
            else
                offsetK = 0;
            end
            % Bremsen
            tBB(1:nZyklen) = linspace(-tvMax,0,nZyklen);%-(nZyklen)*dt+dt:dt:0;

            sB(1:nZyklen) = -sign(zielPosition-startPosition) *  1/2 * aMax * tBB(1:nZyklen).^2 + sA(nZyklen-offset)+sK(nZyklenK-offsetK);
            vB(1:nZyklen) = -sign(zielPosition-startPosition) *  aMax * tBB(1:nZyklen);
            s(1:2*nZyklen+nZyklenK) = [sA(1:nZyklen) sK(1:nZyklenK) sB(1:nZyklen)]+startPosition;
            v(1:2*nZyklen+nZyklenK) = [vA(1:nZyklen) vK(1:nZyklenK) vB(1:nZyklen)];
         end
        firstRun = 0;
    end
    % Ausgabe
    sollPosition = s(n);
    sollGeschwindigkeit = v(n);
    if n < (2*nZyklen+nZyklenK-1)
        n = n + 1;
         fertig = 0;
     elseif nZyklen == nGr || nZyklenK == nGr 
         fertig = 1;
    end

== stateflow chart Gesamt/Regelung1/Zustandsautomat/FertigunsbereichsLogik ==
  state Hauptding [parallel]
    settings: executionOrder=1
    state Warten
      entry: ZielAnfordern = 1;
      exit: ZielAnfordern = 0;
    state Neues_Ziel_erhalten
    note: => Greifer öffnen
    note: => Warten
    note: => Greifer schließen
    state Vorposition_nach_FachAnfahrt
      entry: StationsNr = letztesZiel + 5;
    state Vorposition_vor_FachAnfahrt
      entry: StationsNr = Ziel + 5;
    state Ziel_anfahren
      entry: StationsNr = Ziel;
    state Station_anfahren
      entry: enable = 1,
      Neue_Planung =1;
    state Station_erreicht
      entry: enable = 1,
      Neue_Planung = 0;
      exit: letztesZiel = StationsNr;
    (default) -> Warten
    Warten -> Warten [order 2] : [Ziel == 999]/{letztesZiel = 999}
    Station_erreicht -> Warten [order 3] : [AktionAnZiel == 2]...
        | /{GreiferPose = 0}
    Station_erreicht -> Warten [order 4]
    Station_erreicht -> Warten [order 2] : [AktionAnZiel == 1] ...
        | /{GreiferPose =1}
    Warten -> Neues_Ziel_erhalten [order 1] : [Ziel ~= letztesZiel]
    Station_erreicht -> Neues_Ziel_erhalten [order 1] : [StationsNr ~= Ziel]
    Neues_Ziel_erhalten -> Vorposition_nach_FachAnfahrt [order 1] : [istEinFach(letztesZiel)]
    Neues_Ziel_erhalten -> Vorposition_vor_FachAnfahrt [order 2] : [istEinFach(Ziel) &&  ...
        |  ~istVorpositionDesFachs(Ziel, letztesZiel)]
    Neues_Ziel_erhalten -> Ziel_anfahren [order 3]
    Station_anfahren -> Vorposition_vor_FachAnfahrt [order 3] : [istEinFach(StationsNr) &&  ...
        | after(2.5/dt, tick)]/{Neue_Planung = 0;korrektur = korrektur+1}
    Ziel_anfahren -> Station_anfahren
    Vorposition_nach_FachAnfahrt -> Station_anfahren
    Vorposition_vor_FachAnfahrt -> Station_anfahren
    Station_anfahren -> Station_erreicht [order 2] : [istEinFach(StationsNr) &&  ...
        | TasterGreifer]
        | /{korrektur = 0}
    Station_anfahren -> Station_erreicht [order 1] : [~istEinFach(StationsNr) &&  ...
        | zielPositionErreicht]
  state Greifer [parallel]
    settings: executionOrder=2
    state GreiferAuf
      entry: GreiferPose=0;
    state GreiferZu
      entry: GreiferPose=1;
    (default) -> GreiferAuf : [LSG == 0]
    GreiferAuf -> GreiferZu : [GreiferPose == 1]
    GreiferZu -> GreiferAuf : [GreiferPose == 0 || LSG==0]
  data: ziel function_input double; antwort function_output double; Ziel function_input double; letztesZiel function_input double; antwort function_output double; Ziel input double; AktionAnZiel input double; ZielAnfordern output double =0; letztesZiel local double =0; enable output double =0; GreiferPose output double; zielPositionErreicht input; StationsNr output double =0; korrektur output double =0; Neue_Planung output double; LSG input double; TasterGreifer input double; dt parameter
  function antwort = istEinFach(ziel):
    | function antwort = istEinFach(ziel)
    |  
    |     if 0 < mod(ziel, 10) &&  mod(ziel, 10) < 4
    |         antwort = 1;
    |     else
    |         antwort = 0;
    |     end
    | 
    | end
  function antwort = istVorpositionDesFachs(Ziel, letztesZiel):
    | function antwort = istVorpositionDesFachs(Ziel, letztesZiel)
    | 
    |     if (letztesZiel - 5) == Ziel
    |         % Fachnummer + 5 = Nummer der Vorposition
    |         antwort = 1;
    |     else
    |         antwort = 0;
    |     end
    | 
    | end

== matlab function Gesamt/Regelung1/Zustandsautomat/KoordonatenTafel1 ==
  data: stationsNr input; zielX output; zielY output; zielPsi output; toleranzStufe output; StationsKoordinaten parameter; enable output; Korrektur input
function [zielX, zielY, zielPsi, toleranzStufe, enable] = koordinaten(stationsNr,StationsKoordinaten,Korrektur)

xBuchtOffset = 10;
% 1 -> genau, 2 -> ungenau
toleranzStufe = 1;
enable = 1;

% Batteriestationen anfahren

if stationsNr == 80
    zielX   = StationsKoordinaten(1,stationsNr);
    zielY   = StationsKoordinaten(2,stationsNr);
    zielPsi = pi;
    return
end

if stationsNr == 90
    zielX   = StationsKoordinaten(1,stationsNr);
    zielY   = StationsKoordinaten(2,stationsNr);
    zielPsi = pi;
    return
end

if stationsNr == 100
    zielX   = StationsKoordinaten(1,stationsNr);
    zielY   = StationsKoordinaten(2,stationsNr);
    zielPsi = pi;
    return
end

if stationsNr == 110
    zielX   = StationsKoordinaten(1,stationsNr);
    zielY   = StationsKoordinaten(2,stationsNr);
    zielPsi = pi;
    return
end

% Warteposition vorne
if mod(stationsNr, 10) == 0 
    toleranzStufe = 2;
    
        % WartePosition 0
        if stationsNr == 0
            %weil Matlab leider nicht von 0 aus zählen kann müssen wir das von
            %Hand abfangen...doofes Matlab
            zielX   = 853;
            zielY   = 2288;
            zielPsi = pi/2;
        else
            zielX   = StationsKoordinaten(1,stationsNr);
            zielY   = StationsKoordinaten(2,stationsNr);
            zielPsi = pi/2;
        end

% Stations-Bucht
elseif 0 < mod(stationsNr, 10) && mod(stationsNr, 10) < 4
    
    zielX   = StationsKoordinaten(1,stationsNr);
    zielY   = StationsKoordinaten(2,stationsNr);
    
    % auf welcher Seite der Station?
    if mod(stationsNr, 20) < 10
        % links
        zielX = zielX + xBuchtOffset+Korrektur *5;
        zielPsi = 0;
    else
        % rechts
        zielX = zielX - xBuchtOffset-Korrektur *5;
        zielPsi = pi;
    end

% Warteposition hinten
elseif mod(stationsNr, 10) == 4
    toleranzStufe = 2;
    
    zielX   = StationsKoordinaten(1,stationsNr);
    zielY   = StationsKoordinaten(2,stationsNr);
    zielPsi = pi/2;

% Warteposition mitte
elseif mod(stationsNr, 10) == 5
    
    zielX   = StationsKoordinaten(1,stationsNr);
    zielY   = StationsKoordinaten(2,stationsNr);
    zielPsi = pi/2;

% Vorposition der Bucht
elseif 5 < mod(stationsNr, 10) && mod(stationsNr, 10) < 9
    
    % auf welcher Seite der Station?
    if mod(stationsNr, 20) < 10
        % links
        zielX   = StationsKoordinaten(1,stationsNr-5) - 100;
        zielY   = StationsKoordinaten(2,stationsNr-5);
        zielPsi = 0;
    else
        % rechts
        zielX   = StationsKoordinaten(1,stationsNr-5) + 100;
        zielY   = StationsKoordinaten(2,stationsNr-5);
        zielPsi = pi;
    end

% eine nicht zugeteilte Stationsnummer wird angefordert
else
    % Roboter anhalten
    enable = 0;

    zielX   = 0;
    zielY   = 0;
    zielPsi = 0;
end

== matlab function Gesamt/Regelung1/Zustandsautomat/zielErreicht ==
  data: roboX input; erreicht output; roboY input; roboPsi input; zielX input; zielY input; zielPsi input; toleranzStufe input
 function erreicht = zielErreicht(roboX, roboY, roboPsi, zielX, zielY, zielPsi, toleranzStufe)

 if( toleranzStufe == 2)
    % ungenau
    transToleranz = 50;
    rotToleranz = pi/2;
 else
    % default = genau
    transToleranz = 15;
    rotToleranz = pi/20;
 end

    erreicht = 0;
    
%     if( TasterGreifer == 1)
%         erreicht = 1;
%         return;
%     end
    
    if( abs(zielX-roboX) > transToleranz)
        return;
    end 
    
    if( abs(zielY-roboY) > transToleranz)
        return;
    end 
       
    if( abs(zielPsi-mod(roboPsi,2*pi)) > rotToleranz)
        return;
    end   

    erreicht = 1;

end
